simulink model "stepRecovery"  (Simulink 8.8)
settings: Solver=FixedStepDiscrete  StartTime=0.0  StopTime="CONFIG.SIMULATION_TIME "  FixedStep=CONFIG.Ts  RelTol=1e-3
InitFcn:
  | cd(fileparts(which(bdroot)));
  | initStepRecovery;
undefined symbols (not defined in the file or in its folder): bVectorConstraints, bVectorConstraintsMPC, CONFIG, ConstraintsMatrix, ConstraintsMatrixMPC, DiscIntNeverNeededParam, gain, mpc_init, reg, ROBOT_DOF, ROBOT_DOF_FOR_SIMULINK, sat, sm, WBT_robotName
libraries: WBToolboxLibrary x112, simulink x13, simulink_extras x4
(part 2 of 4)

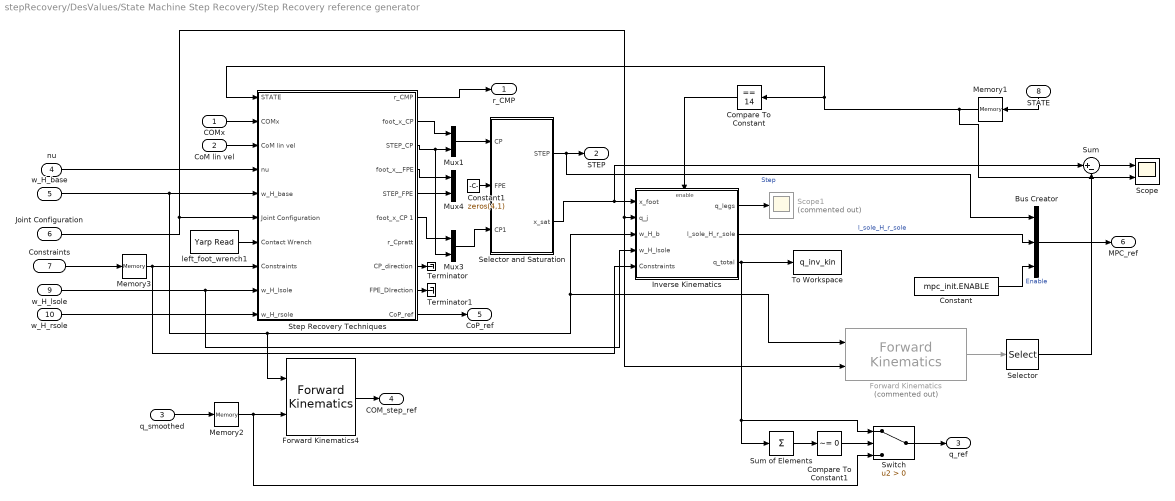
== system stepRecovery/DesValues/State Machine Step Recovery/Step Recovery reference generator ==
  COMx : Inport
  CoM lin vel : Inport  Port=2
  "q_smoothed " : Inport  Port=3
  nu : Inport  Port=4
  w_H_base : Inport  Port=5
  Joint Configuration : Inport  Port=6
  Constraints : Inport  Port=7
  STATE : Inport  Port=8
  w_H_lsole : Inport  Port=9
  w_H_rsole : Inport  Port=10
  Bus Creator : BusCreator  Inputs=3
  Compare To Constant : simulink/Logic and Bit Operations/Compare To Constant  relop===  const=14  OutDataTypeStr=boolean
  Compare To Constant1 : simulink/Logic and Bit Operations/Compare To Constant  relop=~=  const=0  OutDataTypeStr=boolean
  Constant : Constant  Value=mpc_init.ENABLE
  Constant1 : Constant  Value=zeros(4,1)
  Forward Kinematics : WBToolboxLibrary/wholeBodyModel/Kinematics/Forward Kinematics  Commented=on  frameName='r_sole'  robotName=WBT_robotName  localName=WBT_modelName  wbiFile=WBT_wbiFilename  wbiList=WBT_wbiList
  Forward Kinematics4 : WBToolboxLibrary/wholeBodyModel/Kinematics/Forward Kinematics  frameName='com'  robotName=WBT_robotName  localName=WBT_modelName  wbiFile=WBT_wbiFilename  wbiList=WBT_wbiList
  Inverse Kinematics : Subsystem  TreatAsAtomicUnit=on
  Memory1 : Memory  X0=2
  Memory2 : Memory
  Memory3 : Memory  X0=[1;1]
  Mux1 : Mux  Inputs=2
  Mux3 : Mux  Inputs=2
  Mux4 : Mux  Inputs=2
  Scope : Scope  NumInputPorts=2
  Scope1 : Scope  Commented=on
  Selector : Selector  NumberOfDimensions=2  InputPortWidth=3  IndexOptions=Index vector (dialog),Index vector (dialog)  Indices=[1:3],4  OutputSizes=1,1
  Selector and Saturation : Subsystem
  "Step Recovery Techniques " : Subsystem
  Sum : Sum  Inputs=|+-
  Sum of Elements : Sum  Inputs=+
  Switch : Switch  Criteria=u2 > Threshold
  Terminator : Terminator
  Terminator1 : Terminator
  To Workspace : ToWorkspace  VariableName=q_inv_kin  SampleTime=-1
  left_foot_wrench1 : WBToolboxLibrary/Utilities/Yarp Read  portName=PORTS.WBDT_LEFTLEG_EE  signalSize=6  blocking=off  timestamp=off  autoconnect=on  errorOnConnection=on
  r_CMP : Outport
  STEP : Outport  Port=2
  q_ref : Outport  Port=3
  COM_step_ref : Outport  Port=4
  CoP_ref : Outport  Port=5
  MPC_ref : Outport  Port=6
  wires:
  nu/1 -> "Step Recovery Techniques "/4(nu)
  Constraints/1 -> Memory3/1
  Joint Configuration/1 -> Forward Kinematics/2, Inverse Kinematics/2(q_j), "Step Recovery Techniques "/6(Joint Configuration)
  STATE/1 -> Memory1/1
  w_H_base/1 -> Forward Kinematics4/1, Forward Kinematics/1, Inverse Kinematics/3(w_H_b), "Step Recovery Techniques "/5(w_H_base)
  Selector and Saturation/1(STEP) -> Bus Creator/1, STEP/1  "Step"
  left_foot_wrench1/1 -> "Step Recovery Techniques "/7(Contact Wrench)
  "Step Recovery Techniques "/1(r_CMP) -> r_CMP/1
  Selector and Saturation/2(x_sat) -> Sum/1, Inverse Kinematics/1(x_foot)
  Inverse Kinematics/1(q_legs) -> Scope1/1
  Compare To Constant/1 -> Inverse Kinematics/Enable
  Memory1/1 -> Scope/2, "Step Recovery Techniques "/1(STATE), Compare To Constant/1
  Forward Kinematics/1 -> Selector/1
  Selector/1 -> Sum/2
  Sum/1 -> Scope/1
  Inverse Kinematics/3("q_total ") -> Switch/1, Sum of Elements/1, To Workspace/1
  "q_smoothed "/1 -> Memory2/1
  Memory2/1 -> Switch/3, Forward Kinematics4/2
  Memory3/1 -> Inverse Kinematics/5(Constraints), "Step Recovery Techniques "/8("Constraints ")
  "Step Recovery Techniques "/3(STEP_CP) -> Mux3/2, Mux1/2
  "Step Recovery Techniques "/2("foot_x_CP ") -> Mux1/1
  "Step Recovery Techniques "/6(foot_x_CP 1) -> Mux3/1
  Mux1/1 -> Selector and Saturation/1(CP)
  Mux3/1 -> Selector and Saturation/3("CP1 ")
  "Step Recovery Techniques "/4(foot_x__FPE) -> Mux4/1
  "Step Recovery Techniques "/5(STEP_FPE) -> Mux4/2
  "Step Recovery Techniques "/8(CP_direction) -> Terminator/1
  "Step Recovery Techniques "/9(FPE_DIrection) -> Terminator1/1
  w_H_lsole/1 -> "Step Recovery Techniques "/9(w_H_lsole), Inverse Kinematics/4(w_H_lsole)
  w_H_rsole/1 -> "Step Recovery Techniques "/10(w_H_rsole)
  COMx/1 -> "Step Recovery Techniques "/2(COMx)
  CoM lin vel/1 -> "Step Recovery Techniques "/3(CoM lin vel)
  Constant1/1 -> Selector and Saturation/2(FPE)
  "Step Recovery Techniques "/10("CoP_ref ") -> CoP_ref/1
  Inverse Kinematics/2(l_sole_H_r_sole) -> Bus Creator/2  "l_sole_H_r_sole"
  Bus Creator/1 -> MPC_ref/1
  Constant/1 -> Bus Creator/3  "Enable"
  Forward Kinematics4/1 -> COM_step_ref/1
  Sum of Elements/1 -> Compare To Constant1/1
  Switch/1 -> q_ref/1
  Compare To Constant1/1 -> Switch/2

== system stepRecovery/DesValues/State Machine Step Recovery/Switch ==
  Constant : Constant  Value=0
  Constant2 : Constant
  Manual Switch : ManualSwitch
  Out1 : Outport
  wires:
  Constant2/1 -> Manual Switch/2
  Manual Switch/1 -> Out1/1
  Constant/1 -> Manual Switch/1

== system stepRecovery/DesValues/State Machine Step Recovery/Visualise external wrenches   ==
  wL_WBDT : Inport
  wR_WBDT : Inport  Port=2
  CHEST_WBDT : Inport  Port=3
  Enable : EnablePort
  Constant : Constant  Value=sm.wrench.thresholdContactOn
  Constant2 : Constant  Value=sm.wrench.thresholdContactOff
  Selector : Selector  Commented=through  InputPortWidth=6  IndexOptions=Index vector (dialog)  Indices=[1:3]  OutputSizes=1
  To Workspace : ToWorkspace  VariableName=left_wrench  SampleTime=-1
  To Workspace1 : ToWorkspace  VariableName=right_wrench  SampleTime=-1
  To Workspace2 : ToWorkspace  VariableName=torso_wrench  SampleTime=-1
  chest ext wrench1 : Scope
  left foot ext wrench : Scope  NumInputPorts=3
  right foot ext wrench : Scope  NumInputPorts=3
  wires:
  Constant2/1 -> right foot ext wrench/3, left foot ext wrench/3  "thresholdContactOff"
  wL_WBDT/1 -> To Workspace/1, left foot ext wrench/1  "wL_WBDT"
  wR_WBDT/1 -> To Workspace1/1, right foot ext wrench/1  "wR_WBDT"
  Constant/1 -> right foot ext wrench/2, left foot ext wrench/2  "thresholdContactOn"
  CHEST_WBDT/1 -> To Workspace2/1, Selector/1
  Selector/1 -> chest ext wrench1/1

== system stepRecovery/DesValues/State Machine Step Recovery/Visualize hom transf5 ==
  "State " : Inport
  H : Inport  Port=2
  "CoM6D ->  CoMXYZ1" : Selector  NumberOfDimensions=2  InputPortWidth=7  IndexOptions=Index vector (dialog),Index vector (dialog)  Indices=[1 2 3],[1 2 3]  OutputSizes=1,1
  Hom : Scope  NumInputPorts=2
  MATLAB Function : MATLAB Function  TreatAsAtomicUnit=on
  p : Scope  NumInputPorts=2
  position : Selector  NumberOfDimensions=2  InputPortWidth=7  IndexOptions=Index vector (dialog),Index vector (dialog)  Indices=[1 2 3],[4]  OutputSizes=1,1
  rollPitchYaw : Scope  NumInputPorts=2
  wires:
  MATLAB Function/1(rollPitchYaw) -> rollPitchYaw/1  "rollPitchYaw"
  "CoM6D ->  CoMXYZ1"/1 -> MATLAB Function/1(R)
  H/1 -> "CoM6D ->  CoMXYZ1"/1, Hom/1, position/1  "H"
  position/1 -> p/1  "position"
  "State "/1 -> Hom/2, rollPitchYaw/2, p/2

== system stepRecovery/DesValues/State Machine Step Recovery/nu ==
  qj : Inport
  w_H_b : Inport  Port=2
  "constraints " : Inport  Port=3
  Get Estimate : WBToolboxLibrary/wholeBodyStates/Get Estimate  estimateType=Joints Velocity  robotName=WBT_robotName  localName=WBT_modelName  wbiFile=WBT_wbiFilename  wbiList=WBT_wbiList
  Jacobian l_sole : WBToolboxLibrary/wholeBodyModel/Jacobians/Jacobian  frameName='l_sole'  robotName=WBT_robotName  localName=WBT_modelName  wbiFile=WBT_wbiFilename  wbiList=WBT_wbiList
  Jacobian r_sole : WBToolboxLibrary/wholeBodyModel/Jacobians/Jacobian  frameName='r_sole'  robotName=WBT_robotName  localName=WBT_modelName  wbiFile=WBT_wbiFilename  wbiList=WBT_wbiList
  MATLAB Function : MATLAB Function  TreatAsAtomicUnit=on
  Mux : Mux  Inputs=2
  vb + Dqj : Outport
  wires:
  w_H_b/1 -> Jacobian l_sole/1, Jacobian r_sole/1
  qj/1 -> Jacobian l_sole/2, Jacobian r_sole/2
  Jacobian l_sole/1 -> MATLAB Function/1(JcLeftFoot)
  MATLAB Function/1(y) -> Mux/1
  "constraints "/1 -> MATLAB Function/3(activeFeetConstraints)
  Jacobian r_sole/1 -> MATLAB Function/2(JcRightFoot)
  Mux/1 -> vb + Dqj/1
  Get Estimate/1 -> Mux/2, MATLAB Function/4(qD)

== system stepRecovery/DesValues/State Machine Step Recovery/visualise inertial ==
  jointAngles : Inport
  inertial : Inport  Port=2
  Enable : EnablePort
  Inv\* : Product  Inputs=/*  Multiplication=Matrix(*)
  Inv\*1 : Product  Inputs=/*  Multiplication=Matrix(*)
  Visualize hom transf1 : Subsystem
  Visualize hom transf2 : Subsystem
  Visualize hom transf3 : Subsystem
  Visualize hom transf4 : Subsystem
  Visualize hom transf5 : Subsystem
  Visualize hom transf6 : Subsystem
  "inertial -> rpy" : Selector  InputPortWidth=12  IndexOptions=Index vector (dialog)  Indices=[1 2 3]  OutputSizes=1
  l_sole_H_root_link2 : Subsystem  mask{link_name='l_sole'}
  l_sole_H_root_link3 : Subsystem  mask{link_name='r_sole'}
  rpy : Scope
  w_H_root_link1 : Subsystem  mask{link_name='r_sole'}
      mask prompts: link_name "link name"
      mask help:
      | This block evaluates the homogeneous transformation between the world and the root link, i.e. ^wH_b. It assumes that the link specified by the variable 'link_name' has a constant position
      | w.r.t. an inertial frame, but it can rotate arbitrarily. This rotation is retrived from the IMU sensor.
      mask Display:
      | str = strrep(link_name, '_','\_');
      | port_label('output',1,['{}^{',str '}H_{root}'],'texmode','on')
      | clear str;
      | 
      | port_label('input',1,'q_j','texmode','on')
      | 
      | port_label('input',2,'inertial','texmode','on')
  w_H_root_link4 : Subsystem  mask{link_name='l_sole'}
      mask prompts: link_name "link name"
      mask help:
      | This block evaluates the homogeneous transformation between the world and the root link, i.e. ^wH_b. It assumes that the link specified by the variable 'link_name' has a constant position
      | w.r.t. an inertial frame, but it can rotate arbitrarily. This rotation is retrived from the IMU sensor.
      mask Display:
      | str = strrep(link_name, '_','\_');
      | port_label('output',1,['{}^{',str '}H_{root}'],'texmode','on')
      | clear str;
      | 
      | port_label('input',1,'q_j','texmode','on')
      | 
      | port_label('input',2,'inertial','texmode','on')
  wires:
  w_H_root_link1/1(w_H_root) -> Inv\*1/2, Visualize hom transf3/1(H)
  Inv\*1/1 -> Visualize hom transf1/1(H)
  l_sole_H_root_link3/1(link_name_H_root_link) -> Inv\*1/1, Visualize hom transf2/1(H)  "r_sole_H_root_link"
  "inertial -> rpy"/1 -> rpy/1
  w_H_root_link4/1(w_H_root) -> Inv\*/2, Visualize hom transf4/1(H)
  Inv\*/1 -> Visualize hom transf5/1(H)
  l_sole_H_root_link2/1(link_name_H_root_link) -> Inv\*/1, Visualize hom transf6/1(H)  "l_sole_H_root_link"
  jointAngles/1 -> l_sole_H_root_link3/1(qj), w_H_root_link1/1(qj), w_H_root_link4/1(qj), l_sole_H_root_link2/1(qj)
  inertial/1 -> w_H_root_link4/2(inertial), w_H_root_link1/2(inertial), "inertial -> rpy"/1

== system stepRecovery/DesValues/State Machine Step Recovery/w_H_root_link1 ==
  qj : Inport
  inertial : Inport  Port=2
  "CoM6D ->  CoMXYZ1" : Selector  NumberOfDimensions=2  InputPortWidth=7  IndexOptions=Index vector (dialog),Index vector (dialog)  Indices=[1 2 3],[1 2 3]  OutputSizes=1,1
  Constant : Constant  Value=zeros(3,1)
  Constant2 : Constant  Value=eye(4)
  Constant5 : Constant  Value=eye(4)
  Constant6 : Constant  Value=eye(4)
  Gain : Gain  Gain=pi/180
  Head state : WBToolboxLibrary/Utilities/Yarp Read  portName=[WBT_robotName, '/head/state:o']  signalSize=6  blocking=off  timestamp=off  autoconnect=on  errorOnConnection=off
  Inv\* : Product  Inputs=/*  Multiplication=Matrix(*)
  Inv\*1 : Product  Inputs=/*  Multiplication=Matrix(*)
  Inv\*2 : Product  Inputs=/  Multiplication=Matrix(*)
  Product : Product  Multiplication=Matrix(*)
  Selector : Selector  InputPortWidth=12  IndexOptions=Index vector (dialog)  Indices=[4 5 6 ]  OutputSizes=1
  Selector1 : Selector  InputPortWidth=6  IndexOptions=Index vector (dialog)  Indices=[1:3]  OutputSizes=1
  Switch : Switch  Criteria=u2 > Threshold
  Switch6 : Switch  Criteria=u2 > Threshold
  USE_IMU4EST_BASE : Constant  Value=CONFIG.USE_IMU4EST_BASE
  USE_IMU4EST_BASE1 : Constant  Value=CONFIG.CORRECT_NECK_IMU
  fromImuToHomogeousTransformFCN : MATLAB Function  TreatAsAtomicUnit=on
  holder 1 : WBToolboxLibrary/Utilities/holder 
  holder 2 : WBToolboxLibrary/Utilities/holder 
  imu : WBToolboxLibrary/wholeBodyModel/Kinematics/Forward Kinematics  frameName='imu_frame'  robotName=WBT_robotName  localName=WBT_modelName  wbiFile=WBT_wbiFilename  wbiList=WBT_wbiList
  l_sole_acc : Scope
  link : WBToolboxLibrary/wholeBodyModel/Kinematics/Forward Kinematics  frameName=link_name  robotName=WBT_robotName  localName=WBT_modelName  wbiFile=WBT_wbiFilename  wbiList=WBT_wbiList
  root_link : WBToolboxLibrary/wholeBodyModel/Kinematics/Forward Kinematics  frameName='root_link'  robotName=WBT_robotName  localName=WBT_modelName  wbiFile=WBT_wbiFilename  wbiList=WBT_wbiList
  w_H_root : Outport
  wires:
  Constant/1 -> Switch/3
  Gain/1 -> Selector1/1
  Switch/1 -> fromImuToHomogeousTransformFCN/6(neck)
  USE_IMU4EST_BASE1/1 -> Switch/2
  Selector1/1 -> Switch/1  "neck"
  Head state/1 -> Gain/1
  Product/1 -> l_sole_acc/1
  Selector/1 -> Product/2  "imu_acce"
  "CoM6D ->  CoMXYZ1"/1 -> Product/1  "l_sole_R_imu"
  Inv\*2/1 -> "CoM6D ->  CoMXYZ1"/1
  holder 2/1 -> fromImuToHomogeousTransformFCN/4(inertial_0)
  holder 1/1 -> fromImuToHomogeousTransformFCN/2(imu_H_link_0)
  root_link/1 -> Inv\*1/2
  qj/1 -> imu/2, link/2, root_link/2
  Constant2/1 -> root_link/1
  fromImuToHomogeousTransformFCN/1(w_H_root) -> Switch6/1
  USE_IMU4EST_BASE/1 -> Switch6/2
  Switch6/1 -> w_H_root/1
  inertial/1 -> fromImuToHomogeousTransformFCN/5(inertial), holder 2/1, Selector/1
  link/1 -> Inv\*1/1, Inv\*/2
  Inv\*1/1 -> fromImuToHomogeousTransformFCN/3(link_H_root), Switch6/3  "link_H_root"
  Constant6/1 -> link/1
  imu/1 -> Inv\*/1
  Inv\*/1 -> fromImuToHomogeousTransformFCN/1(imu_H_link), holder 1/1, Inv\*2/1  "imu_H_link"
  Constant5/1 -> imu/1

== system stepRecovery/DesValues/State Machine Step Recovery/w_H_root_link4 ==
  qj : Inport
  inertial : Inport  Port=2
  "CoM6D ->  CoMXYZ1" : Selector  NumberOfDimensions=2  InputPortWidth=7  IndexOptions=Index vector (dialog),Index vector (dialog)  Indices=[1 2 3],[1 2 3]  OutputSizes=1,1
  Constant : Constant  Value=zeros(3,1)
  Constant2 : Constant  Value=eye(4)
  Constant5 : Constant  Value=eye(4)
  Constant6 : Constant  Value=eye(4)
  Gain : Gain  Gain=pi/180
  Head state : WBToolboxLibrary/Utilities/Yarp Read  portName=[WBT_robotName, '/head/state:o']  signalSize=6  blocking=off  timestamp=off  autoconnect=on  errorOnConnection=off
  Inv\* : Product  Inputs=/*  Multiplication=Matrix(*)
  Inv\*1 : Product  Inputs=/*  Multiplication=Matrix(*)
  Inv\*2 : Product  Inputs=/  Multiplication=Matrix(*)
  Product : Product  Multiplication=Matrix(*)
  Selector : Selector  InputPortWidth=12  IndexOptions=Index vector (dialog)  Indices=[4 5 6 ]  OutputSizes=1
  Selector1 : Selector  InputPortWidth=6  IndexOptions=Index vector (dialog)  Indices=[1:3]  OutputSizes=1
  Switch : Switch  Criteria=u2 > Threshold
  Switch6 : Switch  Criteria=u2 > Threshold
  USE_IMU4EST_BASE : Constant  Value=CONFIG.USE_IMU4EST_BASE
  USE_IMU4EST_BASE1 : Constant  Value=CONFIG.CORRECT_NECK_IMU
  fromImuToHomogeousTransformFCN : MATLAB Function  TreatAsAtomicUnit=on
  holder 1 : WBToolboxLibrary/Utilities/holder 
  holder 2 : WBToolboxLibrary/Utilities/holder 
  imu : WBToolboxLibrary/wholeBodyModel/Kinematics/Forward Kinematics  frameName='imu_frame'  robotName=WBT_robotName  localName=WBT_modelName  wbiFile=WBT_wbiFilename  wbiList=WBT_wbiList
  l_sole_acc : Scope
  link : WBToolboxLibrary/wholeBodyModel/Kinematics/Forward Kinematics  frameName=link_name  robotName=WBT_robotName  localName=WBT_modelName  wbiFile=WBT_wbiFilename  wbiList=WBT_wbiList
  root_link : WBToolboxLibrary/wholeBodyModel/Kinematics/Forward Kinematics  frameName='root_link'  robotName=WBT_robotName  localName=WBT_modelName  wbiFile=WBT_wbiFilename  wbiList=WBT_wbiList
  w_H_root : Outport
  wires:
  Constant/1 -> Switch/3
  Gain/1 -> Selector1/1
  Switch/1 -> fromImuToHomogeousTransformFCN/6(neck)
  USE_IMU4EST_BASE1/1 -> Switch/2
  Selector1/1 -> Switch/1  "neck"
  Head state/1 -> Gain/1
  Product/1 -> l_sole_acc/1
  Selector/1 -> Product/2  "imu_acce"
  "CoM6D ->  CoMXYZ1"/1 -> Product/1  "l_sole_R_imu"
  Inv\*2/1 -> "CoM6D ->  CoMXYZ1"/1
  holder 2/1 -> fromImuToHomogeousTransformFCN/4(inertial_0)
  holder 1/1 -> fromImuToHomogeousTransformFCN/2(imu_H_link_0)
  root_link/1 -> Inv\*1/2
  qj/1 -> imu/2, link/2, root_link/2
  Constant2/1 -> root_link/1
  fromImuToHomogeousTransformFCN/1(w_H_root) -> Switch6/1
  USE_IMU4EST_BASE/1 -> Switch6/2
  Switch6/1 -> w_H_root/1
  inertial/1 -> fromImuToHomogeousTransformFCN/5(inertial), holder 2/1, Selector/1
  link/1 -> Inv\*1/1, Inv\*/2
  Inv\*1/1 -> fromImuToHomogeousTransformFCN/3(link_H_root), Switch6/3  "link_H_root"
  Constant6/1 -> link/1
  imu/1 -> Inv\*/1
  Inv\*/1 -> fromImuToHomogeousTransformFCN/1(imu_H_link), holder 1/1, Inv\*2/1  "imu_H_link"
  Constant5/1 -> imu/1

== system stepRecovery/DesValues/State Machine Step Recovery/xCom ==
  qj : Inport
  w_H_b : Inport  Port=2
  "CoM6D ->  CoMXYZ2" : Selector  NumberOfDimensions=2  InputPortWidth=7  IndexOptions=Index vector (dialog),Index vector (dialog)  Indices=[1 2 3],[4]  OutputSizes=1,1
  com : WBToolboxLibrary/wholeBodyModel/Kinematics/Forward Kinematics  frameName='com'  robotName=WBT_robotName  localName=WBT_modelName  wbiFile=WBT_wbiFilename  wbiList=WBT_wbiList
  xCom : Outport
  wires:
  w_H_b/1 -> com/1
  com/1 -> "CoM6D ->  CoMXYZ2"/1
  "CoM6D ->  CoMXYZ2"/1 -> xCom/1
  qj/1 -> com/2

== system stepRecovery/DesValues/State Machine Step Recovery/xCom1 ==
  qj : Inport
  w_H_b : Inport  Port=2
  "CoM6D ->  CoMXYZ2" : Selector  NumberOfDimensions=2  InputPortWidth=7  IndexOptions=Index vector (dialog),Index vector (dialog)  Indices=[1 2 3],[4]  OutputSizes=1,1
  com : WBToolboxLibrary/wholeBodyModel/Kinematics/Forward Kinematics  frameName='com'  robotName=WBT_robotName  localName=WBT_modelName  wbiFile=WBT_wbiFilename  wbiList=WBT_wbiList
  xCom : Outport
  wires:
  w_H_b/1 -> com/1
  com/1 -> "CoM6D ->  CoMXYZ2"/1
  "CoM6D ->  CoMXYZ2"/1 -> xCom/1
  qj/1 -> com/2

== system stepRecovery/controller_QP/MPC /omega ==
  COMx : Inport
  Constant : Constant  Value=9.81
  Divide : Product  Inputs=*/
  Selector : Selector  InputPortWidth=3  IndexOptions=Index vector (dialog)  Indices=[3]  OutputSizes=1
  Sqrt : Sqrt  SaturateOnIntegerOverflow=on
  holder 1 : WBToolboxLibrary/Utilities/holder 
  COMz0 : Outport
  omega : Outport  Port=2
  wires:
  COMx/1 -> Selector/1
  Selector/1 -> holder 1/1
  holder 1/1 -> COMz0/1, Divide/2
  Constant/1 -> Divide/1
  Divide/1 -> Sqrt/1
  Sqrt/1 -> omega/1

== system stepRecovery/controller_QP/QP/Subsystem ==
  LEFT_RIGHT_FOOT_IN_CONTACT : Inport
  HessianMatrixQP2Feet : Inport  Port=2
  gradientQP2Feet : Inport  Port=3
  ConstraintsMatrixQP2Feet : Inport  Port=4
  bVectorConstraintsQp2Feet : Inport  Port=5
  USE_QP : Inport  Port=6
  HessianMatrixQP1Foot : Inport  Port=7
  gradientQP1Foot : Inport  Port=8
  ConstraintsMatrixQP1Foot : Inport  Port=9
  bVectorConstraintsQP1Foot : Inport  Port=10
  Enable : EnablePort
  Level-2 MATLAB S-Function : M-S-Function  FunctionName=QpBalancing
  f0TwoFeet : Outport
  ExitFlag : Outport  Port=2
  f0OneFoot : Outport  Port=3
  wires:
  Level-2 MATLAB S-Function/1 -> f0TwoFeet/1
  Level-2 MATLAB S-Function/2 -> ExitFlag/1  "Exit flag QP two feet"
  HessianMatrixQP1Foot/1 -> Level-2 MATLAB S-Function/7
  bVectorConstraintsQP1Foot/1 -> Level-2 MATLAB S-Function/10
  gradientQP1Foot/1 -> Level-2 MATLAB S-Function/8
  ConstraintsMatrixQP1Foot/1 -> Level-2 MATLAB S-Function/9
  Level-2 MATLAB S-Function/3 -> f0OneFoot/1
  LEFT_RIGHT_FOOT_IN_CONTACT/1 -> Level-2 MATLAB S-Function/1
  HessianMatrixQP2Feet/1 -> Level-2 MATLAB S-Function/2
  gradientQP2Feet/1 -> Level-2 MATLAB S-Function/3
  ConstraintsMatrixQP2Feet/1 -> Level-2 MATLAB S-Function/4
  bVectorConstraintsQp2Feet/1 -> Level-2 MATLAB S-Function/5
  USE_QP/1 -> Level-2 MATLAB S-Function/6

== system stepRecovery/controller_QP/QP/Subsystem1 ==
  LEFT_RIGHT_FOOT_IN_CONTACT : Inport
  HessianMatrixQP2Feet : Inport  Port=2
  gradientQP2Feet : Inport  Port=3
  ConstraintsMatrixQP2Feet : Inport  Port=4
  bVectorConstraintsQp2Feet : Inport  Port=5
  USE_QP : Inport  Port=6
  HessianMatrixQP1Foot : Inport  Port=7
  gradientQP1Foot : Inport  Port=8
  ConstraintsMatrixQP1Foot : Inport  Port=9
  bVectorConstraintsQP1Foot : Inport  Port=10
  Enable : EnablePort
  Level-2 MATLAB S-Function : M-S-Function  FunctionName=QpTwoFeetStep
  f0TwoFeet : Outport
  ExitFlag : Outport  Port=2
  f0OneFoot : Outport  Port=3
  slack : Outport  Port=4
  wires:
  USE_QP/1 -> Level-2 MATLAB S-Function/6
  bVectorConstraintsQp2Feet/1 -> Level-2 MATLAB S-Function/5
  ConstraintsMatrixQP2Feet/1 -> Level-2 MATLAB S-Function/4
  gradientQP2Feet/1 -> Level-2 MATLAB S-Function/3
  HessianMatrixQP2Feet/1 -> Level-2 MATLAB S-Function/2
  LEFT_RIGHT_FOOT_IN_CONTACT/1 -> Level-2 MATLAB S-Function/1
  Level-2 MATLAB S-Function/3 -> f0OneFoot/1
  ConstraintsMatrixQP1Foot/1 -> Level-2 MATLAB S-Function/9
  gradientQP1Foot/1 -> Level-2 MATLAB S-Function/8
  bVectorConstraintsQP1Foot/1 -> Level-2 MATLAB S-Function/10
  HessianMatrixQP1Foot/1 -> Level-2 MATLAB S-Function/7
  Level-2 MATLAB S-Function/2 -> ExitFlag/1  "Exit flag QP two feet"
  Level-2 MATLAB S-Function/1 -> f0TwoFeet/1
  Level-2 MATLAB S-Function/4 -> slack/1

== system stepRecovery/controller_QP/QP/Visualize eventual QP failures ==
  exitFlagQP : Inport
  state : Inport  Port=2
  Enable : EnablePort
  "QP status (0: no failure, 1: not using)" : Scope  NumInputPorts=2
  wires:
  exitFlagQP/1 -> "QP status (0: no failure, 1: not using)"/1  "exitFlagQP"
  state/1 -> "QP status (0: no failure, 1: not using)"/2

== system stepRecovery/controller_QP/integralOf Hw/l_sole_H_root_link ==
  qj0 : Inport
  Constant5 : Constant  Value=eye(4)
  Constant6 : Constant  Value=eye(4)
  Inv\* : Product  Inputs=/*  Multiplication=Matrix(*)
  l_sole : WBToolboxLibrary/wholeBodyModel/Kinematics/Forward Kinematics  frameName='l_sole'  robotName=WBT_robotName  localName=WBT_modelName  wbiFile=WBT_wbiFilename  wbiList=WBT_wbiList
  root_link : WBToolboxLibrary/wholeBodyModel/Kinematics/Forward Kinematics  frameName='root_link'  robotName=WBT_robotName  localName=WBT_modelName  wbiFile=WBT_wbiFilename  wbiList=WBT_wbiList
  l_sole_H_root_link : Outport
  wires:
  Constant5/1 -> l_sole/1
  Inv\*/1 -> l_sole_H_root_link/1  "l_sole_H_root_link"
  l_sole/1 -> Inv\*/1
  Constant6/1 -> root_link/1
  qj0/1 -> l_sole/2, root_link/2
  root_link/1 -> Inv\*/2

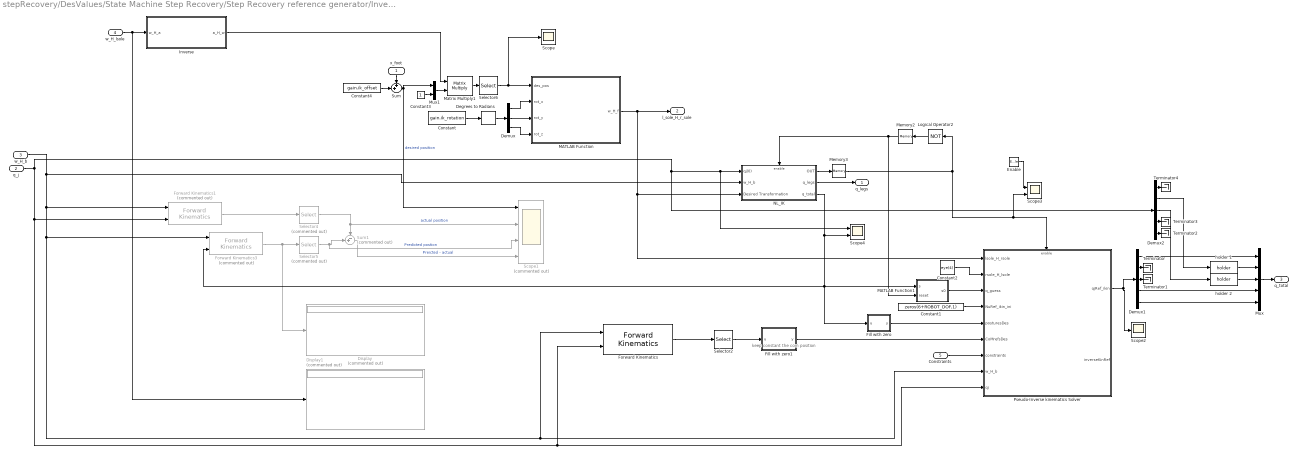
== system stepRecovery/DesValues/State Machine Step Recovery/Step Recovery reference generator/Inverse Kinematics ==
  note: keep constant the com position
  x_foot : Inport
  q_j : Inport  Port=2
  w_H_b : Inport  Port=3
  w_H_lsole : Inport  Port=4
  Constraints : Inport  Port=5
  Enable : EnablePort  ShowOutputPort=on
  Constant : Constant  Value=gain.ik_rotation
  Constant1 : Constant  Value=zeros(6+ROBOT_DOF,1)
  Constant2 : Constant  Value=eye(4)
  Constant3 : Constant
  Constant4 : Constant  Value=gain.ik_offset
  Degrees to Radians : simulink_extras/Transformations/Degrees to Radians
  Demux : Demux  Outputs=3
  Demux1 : Demux  Outputs=[3;4;4;6;6]
  Demux2 : Demux  Outputs=[3;4;4;6;6]
  Display : Display  Commented=on
  Display1 : Display  Commented=on
  Fill with zero : MATLAB Function  TreatAsAtomicUnit=on
  Fill with zero1 : MATLAB Function  TreatAsAtomicUnit=on
  Forward Kinematics : WBToolboxLibrary/wholeBodyModel/Kinematics/Forward Kinematics  frameName='com'  robotName=WBT_robotName  localName=WBT_modelName  wbiFile=WBT_wbiFilename  wbiList=WBT_wbiList
  Forward Kinematics1 : WBToolboxLibrary/wholeBodyModel/Kinematics/Forward Kinematics  Commented=on  frameName='r_sole'  robotName=WBT_robotName  localName=WBT_modelName  wbiFile=WBT_wbiFilename  wbiList=WBT_wbiList
  Forward Kinematics3 : WBToolboxLibrary/wholeBodyModel/Kinematics/Forward Kinematics  Commented=on  frameName='r_sole'  robotName=WBT_robotName  localName=WBT_modelName  wbiFile=WBT_wbiFilename  wbiList=WBT_wbiList
  Inverse : MATLAB Function  TreatAsAtomicUnit=on
  Logical Operator2 : Logic  Operator=NOT  AllPortsSameDT=off  OutDataTypeStr=boolean
  MATLAB Function : MATLAB Function  TreatAsAtomicUnit=on
  MATLAB Function1 : MATLAB Function  TreatAsAtomicUnit=on
  Matrix Multiply1 : Product  Multiplication=Matrix(*)
  Memory2 : Memory  X0=1
  Memory3 : Memory
  Mux : Mux  Inputs=[3;4;4;6;6]
  Mux1 : Mux  Inputs=2
  NL_IK : Subsystem
  Pseudo-Inverse kinematics Solver : Subsystem
  Scope : Scope
  Scope1 : Scope  Commented=on  NumInputPorts=4
  Scope2 : Scope
  Scope3 : Scope  NumInputPorts=2
  Scope4 : Scope  NumInputPorts=2
  Selector2 : Selector  NumberOfDimensions=2  InputPortWidth=3  IndexOptions=Index vector (dialog),Index vector (dialog)  Indices=[1:3],4  OutputSizes=1,1
  Selector4 : Selector  Commented=on  NumberOfDimensions=2  InputPortWidth=4  IndexOptions=Index vector (dialog),Index vector (dialog)  Indices=[1:3],4  OutputSizes=1,1
  Selector5 : Selector  Commented=on  NumberOfDimensions=2  InputPortWidth=4  IndexOptions=Index vector (dialog),Index vector (dialog)  Indices=[1:3],4  OutputSizes=1,1
  Selector6 : Selector  InputPortWidth=4  IndexOptions=Index vector (dialog)  Indices=[1:3]  OutputSizes=1
  Sum : Sum  Inputs=++|
  Sum1 : Sum  Commented=on  Inputs=-+|
  Terminator{,1..4} (5 alike) : Terminator
  holder 1 : WBToolboxLibrary/Utilities/holder 
  holder 2 : WBToolboxLibrary/Utilities/holder 
  q_legs : Outport
  l_sole_H_r_sole : Outport  Port=2
  "q_total " : Outport  Port=3
  wires:
  w_H_lsole/1 -> Display1/1, Inverse/1(w_H_a)
  Inverse/1(a_H_w) -> Matrix Multiply1/1
  Forward Kinematics1/1 -> Selector4/1
  Sum/1 -> Mux1/1, Scope1/1  "desired position"
  Constant4/1 -> Sum/2
  x_foot/1 -> Sum/1
  Forward Kinematics3/1 -> Display/1, Selector5/1
  Selector4/1 -> Sum1/1, Scope1/2  "actual position"
  Sum1/1 -> Scope1/4  "Preicted - actual"
  Mux1/1 -> Matrix Multiply1/2
  Constant3/1 -> Mux1/2
  Selector6/1 -> Scope/1, MATLAB Function/1(des_pos)
  Matrix Multiply1/1 -> Selector6/1
  Selector5/1 -> Scope1/3, Sum1/2  "Predicted postion"
  Constant/1 -> Degrees to Radians/1
  Degrees to Radians/1 -> Demux/1
  Demux/2 -> MATLAB Function/3(rot_y)
  Demux/1 -> MATLAB Function/2(rot_x)
  Demux/3 -> MATLAB Function/4(rot_z)
  MATLAB Function/1(w_H_f) -> l_sole_H_r_sole/1, Pseudo-Inverse kinematics Solver/1("lsole_H_rsole "), NL_IK/3(Desired Transformation)
  w_H_b/1 -> NL_IK/2(w_H_b), Forward Kinematics1/1, Forward Kinematics/1, Pseudo-Inverse kinematics Solver/8("w_H_b "), Forward Kinematics3/1
  Constant1/1 -> Pseudo-Inverse kinematics Solver/4(NuRef_ikin_ini)
  Constraints/1 -> Pseudo-Inverse kinematics Solver/7(constraints)
  Fill with zero1/1(y) -> Pseudo-Inverse kinematics Solver/6(CoMrefsDes)
  Forward Kinematics/1 -> Selector2/1
  Selector2/1 -> Fill with zero1/1(u)
  Fill with zero/1(y) -> Pseudo-Inverse kinematics Solver/5(posturesDes)
  MATLAB Function1/1(s0) -> Pseudo-Inverse kinematics Solver/3(q_guess)
  Logical Operator2/1 -> Memory2/1
  q_j/1 -> Forward Kinematics/2, Pseudo-Inverse kinematics Solver/9(qj), Forward Kinematics1/2, Demux2/1, Scope4/1, NL_IK/1(qj(0))
  Demux1/1 -> Mux/1
  Demux1/4 -> Mux/4
  Demux1/5 -> Mux/5
  Demux1/2 -> Terminator/1
  Demux1/3 -> Terminator1/1
  holder 2/1 -> Mux/3
  holder 1/1 -> Mux/2
  Demux2/2 -> holder 1/1
  Demux2/3 -> holder 2/1
  Demux2/5 -> Terminator2/1
  Demux2/4 -> Terminator3/1
  Demux2/1 -> Terminator4/1
  Memory2/1 -> NL_IK/Enable, MATLAB Function1/2(reset)
  Enable/1 -> Scope3/1
  Memory3/1 -> Pseudo-Inverse kinematics Solver/Enable, Scope3/2, Logical Operator2/1
  Mux/1 -> "q_total "/1
  NL_IK/2(q_legs) -> q_legs/1
  NL_IK/1(OUT) -> Memory3/1
  Constant2/1 -> Pseudo-Inverse kinematics Solver/2(rsole_H_lsole)
  NL_IK/3(q_total) -> Forward Kinematics3/2, MATLAB Function1/1(s), Fill with zero/1(u), Scope4/2
  Pseudo-Inverse kinematics Solver/1(qjRef_ikin) -> Scope2/1, Demux1/1

== system stepRecovery/DesValues/State Machine Step Recovery/Step Recovery reference generator/Selector and Saturation ==
  CP : Inport
  FPE : Inport  Port=2
  "CP1 " : Inport  Port=3
  Constant : Constant  Value=2*sqrt(gain.leg_length^2 - gain.minimum_height^2)
  Constant1 : Constant  Value=gain.min_step_length
  Constant2 : Constant  Value=CONFIG.SR.TECHNIQUE
  Demux : Demux
  Dot Product : DotProduct  InputSameDT=on  OutDataTypeStr=Inherit: Inherit via internal rule
  MATLAB Function : MATLAB Function  TreatAsAtomicUnit=on
  Multiport Switch : MultiPortSwitch  DataPortOrder=Specify indices  DataPortIndices={2,1,0}
  Mux : Mux  Inputs=3
  Mux1 : Mux  Inputs=3
  Scope : Scope  Commented=on  NumInputPorts=4
  Sqrt : Sqrt  SaturateOnIntegerOverflow=on
  To Workspace : ToWorkspace  VariableName=IS_SATURATED  SampleTime=-1
      settings: Save2DSignal=2-D array (concatenate along first dimension)
  STEP : Outport
  x_sat : Outport  Port=2
  wires:
  Mux1/1 -> Scope/4, Dot Product/2, Dot Product/1, MATLAB Function/1(x)  "X"
  Constant/1 -> MATLAB Function/2(max_d), Mux/2  "max module"
  MATLAB Function/1(x_sat) -> Scope/3, x_sat/1  "X_SAT"
  MATLAB Function/2(SAT) -> Scope/1, To Workspace/1  "SAT"
  Mux/1 -> Scope/2  "MODULE"
  Sqrt/1 -> Mux/1  "desired module"
  Dot Product/1 -> Sqrt/1
  Constant1/1 -> Mux/3, MATLAB Function/3(min_d)  "min module"
  Multiport Switch/1 -> Demux/1  "X"
  Demux/4 -> STEP/1
  CP/1 -> Multiport Switch/4  "X"
  FPE/1 -> Multiport Switch/3
  "CP1 "/1 -> Multiport Switch/2
  Constant2/1 -> Multiport Switch/1
  Demux/2 -> Mux1/2
  Demux/3 -> Mux1/3
  Demux/1 -> Mux1/1  "X"

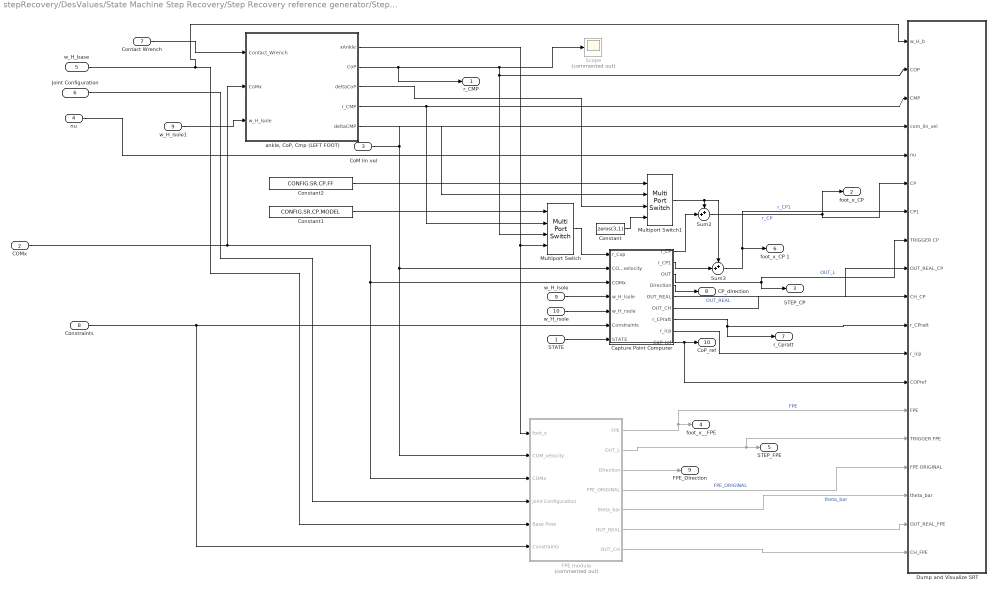
== system stepRecovery/DesValues/State Machine Step Recovery/Step Recovery reference generator/Step Recovery Techniques  ==
  STATE : Inport
  COMx : Inport  Port=2
  CoM lin vel : Inport  Port=3
  nu : Inport  Port=4
  w_H_base : Inport  Port=5
  Joint Configuration : Inport  Port=6
  Contact Wrench : Inport  Port=7
  "Constraints " : Inport  Port=8
  w_H_lsole : Inport  Port=9
  w_H_rsole : Inport  Port=10
  Capture Point Computer : Subsystem
  Constant : Constant  Value=zeros(3,1)
  Constant1 : Constant  Value=CONFIG.SR.CP.MODEL
  Constant2 : Constant  Value=CONFIG.SR.CP.FF
  "Dump and Visualize SRT " : Subsystem
  FPE module : Subsystem  Commented=on
  Multiport Switch : MultiPortSwitch  DataPortOrder=Specify indices  DataPortIndices={2,1,0}
  Multiport Switch1 : MultiPortSwitch  DataPortOrder=Specify indices  DataPortIndices={2,1,0}
  Scope : Scope  Commented=on
  Sum2 : Sum  Inputs=++|
  Sum3 : Sum  Inputs=++|
  "ankle, CoP, Cmp (LEFT FOOT)" : Subsystem
  w_H_lsole1 : InportShadow  Port=9
  r_CMP : Outport
  "foot_x_CP " : Outport  Port=2
  STEP_CP : Outport  Port=3
  foot_x__FPE : Outport  Port=4
  STEP_FPE : Outport  Port=5
  foot_x_CP 1 : Outport  Port=6
  "r_Cpratt " : Outport  Port=7
  CP_direction : Outport  Port=8
  FPE_DIrection : Outport  Port=9
  "CoP_ref " : Outport  Port=10
  wires:
  Joint Configuration/1 -> FPE module/4(Joint Configuration)
  w_H_base/1 -> FPE module/5(Base Pose), "Dump and Visualize SRT "/1(w_H_b)
  FPE module/1(FPE) -> "Dump and Visualize SRT "/14(FPE), foot_x__FPE/1  "FPE"
  Sum2/1 -> "foot_x_CP "/1, "Dump and Visualize SRT "/6(CP)  "r_CP"
  Capture Point Computer/3(OUT) -> "Dump and Visualize SRT "/8(TRIGGER CP), STEP_CP/1  "OUT_L"
  Sum3/1 -> "Dump and Visualize SRT "/7(CP1), foot_x_CP 1/1  "r_CP1"
  FPE module/3(Direction) -> FPE_DIrection/1
  Capture Point Computer/4(Direction) -> CP_direction/1
  Capture Point Computer/1(r_CP) -> Sum2/2
  Capture Point Computer/2(r_CP1) -> Sum3/2
  "Constraints "/1 -> FPE module/6(Constraints), Capture Point Computer/6("Constraints ")
  FPE module/2(OUT_L) -> "Dump and Visualize SRT "/15(TRIGGER FPE), STEP_FPE/1
  CoM lin vel/1 -> "Dump and Visualize SRT "/4(com_lin_vel), FPE module/2(COM_velocity), Capture Point Computer/2(COM velocity)
  COMx/1 -> FPE module/3(COMx), Capture Point Computer/3(COMx), "ankle, CoP, Cmp (LEFT FOOT)"/2(CoMx)
  "ankle, CoP, Cmp (LEFT FOOT)"/2(CoP) -> r_CMP/1, Scope/1, Multiport Switch/3, "Dump and Visualize SRT "/2(COP)
  "ankle, CoP, Cmp (LEFT FOOT)"/1(xAnkle) -> FPE module/1(foot_x), Multiport Switch/4
  Contact Wrench/1 -> "ankle, CoP, Cmp (LEFT FOOT)"/1(Contact_Wrench)
  nu/1 -> "Dump and Visualize SRT "/5(nu)
  "ankle, CoP, Cmp (LEFT FOOT)"/4(r_CMP) -> "Dump and Visualize SRT "/3(CMP), Multiport Switch/2
  Capture Point Computer/5(OUT_REAL) -> "Dump and Visualize SRT "/9(OUT_REAL_CP)  "OUT_REAL"
  Capture Point Computer/6(OUT_CH) -> "Dump and Visualize SRT "/10(CH_CP)
  FPE module/4(FPE_ORIGINAL) -> "Dump and Visualize SRT "/16(FPE ORIGINAL)  "FPE_ORIGINAL"
  FPE module/5(theta_bar) -> "Dump and Visualize SRT "/17(theta_bar)  "theta_bar"
  FPE module/6(OUT_REAL) -> "Dump and Visualize SRT "/18(OUT_REAL_FPE)
  FPE module/7(OUT_CH) -> "Dump and Visualize SRT "/19(CH_FPE)
  Multiport Switch/1 -> Capture Point Computer/1(r_Cxp)
  Multiport Switch1/1 -> Sum3/1, Sum2/1
  Constant/1 -> Multiport Switch1/4
  "ankle, CoP, Cmp (LEFT FOOT)"/3(deltaCoP) -> Multiport Switch1/3
  "ankle, CoP, Cmp (LEFT FOOT)"/5(deltaCMP) -> Multiport Switch1/2
  Constant1/1 -> Multiport Switch/1
  Constant2/1 -> Multiport Switch1/1
  w_H_lsole/1 -> Capture Point Computer/4(w_H_lsole)
  w_H_rsole/1 -> Capture Point Computer/5(w_H_rsole)
  w_H_lsole1/1 -> "ankle, CoP, Cmp (LEFT FOOT)"/3(w_H_lsole)
  STATE/1 -> Capture Point Computer/7(STATE)
  Capture Point Computer/7("r_CPratt ") -> "r_Cpratt "/1, "Dump and Visualize SRT "/11("r_CPratt ")
  Capture Point Computer/8(r_icp) -> "Dump and Visualize SRT "/12(r_icp)
  Capture Point Computer/9(CoP_ref) -> "Dump and Visualize SRT "/13(COPref), "CoP_ref "/1

== system stepRecovery/DesValues/State Machine Step Recovery/visualise inertial/Visualize hom transf1 ==
  H : Inport
  "CoM6D ->  CoMXYZ1" : Selector  NumberOfDimensions=2  InputPortWidth=7  IndexOptions=Index vector (dialog),Index vector (dialog)  Indices=[1 2 3],[1 2 3]  OutputSizes=1,1
  "CoM6D ->  CoMXYZ2" : Selector  NumberOfDimensions=2  InputPortWidth=7  IndexOptions=Index vector (dialog),Index vector (dialog)  Indices=[1 2 3],[4]  OutputSizes=1,1
  Hom : Scope
  MATLAB Function : MATLAB Function  TreatAsAtomicUnit=on
  p : Scope
  rollPitchYaw : Scope
  wires:
  MATLAB Function/1(rollPitchYaw) -> rollPitchYaw/1
  "CoM6D ->  CoMXYZ1"/1 -> MATLAB Function/1(R)
  H/1 -> "CoM6D ->  CoMXYZ1"/1, Hom/1, "CoM6D ->  CoMXYZ2"/1
  "CoM6D ->  CoMXYZ2"/1 -> p/1

== system stepRecovery/DesValues/State Machine Step Recovery/visualise inertial/Visualize hom transf2 ==
  H : Inport
  "CoM6D ->  CoMXYZ1" : Selector  NumberOfDimensions=2  InputPortWidth=7  IndexOptions=Index vector (dialog),Index vector (dialog)  Indices=[1 2 3],[1 2 3]  OutputSizes=1,1
  "CoM6D ->  CoMXYZ2" : Selector  NumberOfDimensions=2  InputPortWidth=7  IndexOptions=Index vector (dialog),Index vector (dialog)  Indices=[1 2 3],[4]  OutputSizes=1,1
  Hom : Scope
  MATLAB Function : MATLAB Function  TreatAsAtomicUnit=on
  p : Scope
  rollPitchYaw : Scope
  wires:
  MATLAB Function/1(rollPitchYaw) -> rollPitchYaw/1
  "CoM6D ->  CoMXYZ1"/1 -> MATLAB Function/1(R)
  H/1 -> "CoM6D ->  CoMXYZ1"/1, Hom/1, "CoM6D ->  CoMXYZ2"/1
  "CoM6D ->  CoMXYZ2"/1 -> p/1

== system stepRecovery/DesValues/State Machine Step Recovery/visualise inertial/Visualize hom transf3 ==
  H : Inport
  "CoM6D ->  CoMXYZ1" : Selector  NumberOfDimensions=2  InputPortWidth=7  IndexOptions=Index vector (dialog),Index vector (dialog)  Indices=[1 2 3],[1 2 3]  OutputSizes=1,1
  "CoM6D ->  CoMXYZ2" : Selector  NumberOfDimensions=2  InputPortWidth=7  IndexOptions=Index vector (dialog),Index vector (dialog)  Indices=[1 2 3],[4]  OutputSizes=1,1
  Hom : Scope
  MATLAB Function : MATLAB Function  TreatAsAtomicUnit=on
  p : Scope
  rollPitchYaw : Scope
  wires:
  MATLAB Function/1(rollPitchYaw) -> rollPitchYaw/1
  "CoM6D ->  CoMXYZ1"/1 -> MATLAB Function/1(R)
  H/1 -> "CoM6D ->  CoMXYZ1"/1, Hom/1, "CoM6D ->  CoMXYZ2"/1
  "CoM6D ->  CoMXYZ2"/1 -> p/1

== system stepRecovery/DesValues/State Machine Step Recovery/visualise inertial/Visualize hom transf4 ==
  H : Inport
  "CoM6D ->  CoMXYZ1" : Selector  NumberOfDimensions=2  InputPortWidth=7  IndexOptions=Index vector (dialog),Index vector (dialog)  Indices=[1 2 3],[1 2 3]  OutputSizes=1,1
  "CoM6D ->  CoMXYZ2" : Selector  NumberOfDimensions=2  InputPortWidth=7  IndexOptions=Index vector (dialog),Index vector (dialog)  Indices=[1 2 3],[4]  OutputSizes=1,1
  Hom : Scope
  MATLAB Function : MATLAB Function  TreatAsAtomicUnit=on
  p : Scope
  rollPitchYaw : Scope
  wires:
  MATLAB Function/1(rollPitchYaw) -> rollPitchYaw/1
  "CoM6D ->  CoMXYZ1"/1 -> MATLAB Function/1(R)
  H/1 -> "CoM6D ->  CoMXYZ1"/1, Hom/1, "CoM6D ->  CoMXYZ2"/1
  "CoM6D ->  CoMXYZ2"/1 -> p/1

== system stepRecovery/DesValues/State Machine Step Recovery/visualise inertial/Visualize hom transf5 ==
  H : Inport
  "CoM6D ->  CoMXYZ1" : Selector  NumberOfDimensions=2  InputPortWidth=7  IndexOptions=Index vector (dialog),Index vector (dialog)  Indices=[1 2 3],[1 2 3]  OutputSizes=1,1
  Hom : Scope
  MATLAB Function : MATLAB Function  TreatAsAtomicUnit=on
  p : Scope
  position : Selector  NumberOfDimensions=2  InputPortWidth=7  IndexOptions=Index vector (dialog),Index vector (dialog)  Indices=[1 2 3],[4]  OutputSizes=1,1
  rollPitchYaw : Scope
  wires:
  MATLAB Function/1(rollPitchYaw) -> rollPitchYaw/1  "rollPitchYaw"
  "CoM6D ->  CoMXYZ1"/1 -> MATLAB Function/1(R)
  H/1 -> "CoM6D ->  CoMXYZ1"/1, Hom/1, position/1  "H"
  position/1 -> p/1  "position"

== system stepRecovery/DesValues/State Machine Step Recovery/visualise inertial/Visualize hom transf6 ==
  H : Inport
  "CoM6D ->  CoMXYZ1" : Selector  NumberOfDimensions=2  InputPortWidth=7  IndexOptions=Index vector (dialog),Index vector (dialog)  Indices=[1 2 3],[1 2 3]  OutputSizes=1,1
  "CoM6D ->  CoMXYZ2" : Selector  NumberOfDimensions=2  InputPortWidth=7  IndexOptions=Index vector (dialog),Index vector (dialog)  Indices=[1 2 3],[4]  OutputSizes=1,1
  Hom : Scope
  MATLAB Function : MATLAB Function  TreatAsAtomicUnit=on
  p : Scope
  rollPitchYaw : Scope
  wires:
  MATLAB Function/1(rollPitchYaw) -> rollPitchYaw/1
  "CoM6D ->  CoMXYZ1"/1 -> MATLAB Function/1(R)
  H/1 -> "CoM6D ->  CoMXYZ1"/1, Hom/1, "CoM6D ->  CoMXYZ2"/1
  "CoM6D ->  CoMXYZ2"/1 -> p/1

== system stepRecovery/DesValues/State Machine Step Recovery/visualise inertial/l_sole_H_root_link2 ==
  qj : Inport
  Constant5 : Constant  Value=eye(4)
  Constant6 : Constant  Value=eye(4)
  Inv\* : Product  Inputs=/*  Multiplication=Matrix(*)
  Visualize hom transf4 : Subsystem
  link_name : WBToolboxLibrary/wholeBodyModel/Kinematics/Forward Kinematics  frameName=link_name  robotName=WBT_robotName  localName=WBT_modelName  wbiFile=WBT_wbiFilename  wbiList=WBT_wbiList
  root_link : WBToolboxLibrary/wholeBodyModel/Kinematics/Forward Kinematics  frameName='root_link'  robotName=WBT_robotName  localName=WBT_modelName  wbiFile=WBT_wbiFilename  wbiList=WBT_wbiList
  link_name_H_root_link : Outport
  wires:
  root_link/1 -> Inv\*/2, Visualize hom transf4/1(H)
  qj/1 -> root_link/2, link_name/2
  Constant6/1 -> root_link/1
  link_name/1 -> Inv\*/1
  Inv\*/1 -> link_name_H_root_link/1  "link_name_H_root_link"
  Constant5/1 -> link_name/1

== system stepRecovery/DesValues/State Machine Step Recovery/visualise inertial/l_sole_H_root_link3 ==
  qj : Inport
  Constant5 : Constant  Value=eye(4)
  Constant6 : Constant  Value=eye(4)
  Inv\* : Product  Inputs=/*  Multiplication=Matrix(*)
  Visualize hom transf4 : Subsystem
  link_name : WBToolboxLibrary/wholeBodyModel/Kinematics/Forward Kinematics  frameName=link_name  robotName=WBT_robotName  localName=WBT_modelName  wbiFile=WBT_wbiFilename  wbiList=WBT_wbiList
  root_link : WBToolboxLibrary/wholeBodyModel/Kinematics/Forward Kinematics  frameName='root_link'  robotName=WBT_robotName  localName=WBT_modelName  wbiFile=WBT_wbiFilename  wbiList=WBT_wbiList
  link_name_H_root_link : Outport
  wires:
  root_link/1 -> Inv\*/2, Visualize hom transf4/1(H)
  qj/1 -> root_link/2, link_name/2
  Constant6/1 -> root_link/1
  link_name/1 -> Inv\*/1
  Inv\*/1 -> link_name_H_root_link/1  "link_name_H_root_link"
  Constant5/1 -> link_name/1

== system stepRecovery/DesValues/State Machine Step Recovery/visualise inertial/w_H_root_link1 ==
  qj : Inport
  inertial : Inport  Port=2
  "CoM6D ->  CoMXYZ1" : Selector  NumberOfDimensions=2  InputPortWidth=7  IndexOptions=Index vector (dialog),Index vector (dialog)  Indices=[1 2 3],[1 2 3]  OutputSizes=1,1
  Constant : Constant  Value=zeros(3,1)
  Constant2 : Constant  Value=eye(4)
  Constant5 : Constant  Value=eye(4)
  Constant6 : Constant  Value=eye(4)
  Gain : Gain  Gain=pi/180
  Head state : WBToolboxLibrary/Utilities/Yarp Read  portName=[WBT_robotName, '/head/state:o']  signalSize=6  blocking=off  timestamp=off  autoconnect=on  errorOnConnection=off
  Inv\* : Product  Inputs=/*  Multiplication=Matrix(*)
  Inv\*1 : Product  Inputs=/*  Multiplication=Matrix(*)
  Inv\*2 : Product  Inputs=/  Multiplication=Matrix(*)
  Product : Product  Multiplication=Matrix(*)
  Selector : Selector  InputPortWidth=12  IndexOptions=Index vector (dialog)  Indices=[4 5 6 ]  OutputSizes=1
  Selector1 : Selector  InputPortWidth=6  IndexOptions=Index vector (dialog)  Indices=[1:3]  OutputSizes=1
  Switch : Switch  Criteria=u2 > Threshold
  Switch6 : Switch  Criteria=u2 > Threshold
  USE_IMU4EST_BASE : Constant  Value=CONFIG.USE_IMU4EST_BASE
  USE_IMU4EST_BASE1 : Constant  Value=CONFIG.CORRECT_NECK_IMU
  fromImuToHomogeousTransformFCN : MATLAB Function  TreatAsAtomicUnit=on
  holder 1 : WBToolboxLibrary/Utilities/holder 
  holder 2 : WBToolboxLibrary/Utilities/holder 
  imu : WBToolboxLibrary/wholeBodyModel/Kinematics/Forward Kinematics  frameName='imu_frame'  robotName=WBT_robotName  localName=WBT_modelName  wbiFile=WBT_wbiFilename  wbiList=WBT_wbiList
  l_sole_acc : Scope
  link : WBToolboxLibrary/wholeBodyModel/Kinematics/Forward Kinematics  frameName=link_name  robotName=WBT_robotName  localName=WBT_modelName  wbiFile=WBT_wbiFilename  wbiList=WBT_wbiList
  root_link : WBToolboxLibrary/wholeBodyModel/Kinematics/Forward Kinematics  frameName='root_link'  robotName=WBT_robotName  localName=WBT_modelName  wbiFile=WBT_wbiFilename  wbiList=WBT_wbiList
  w_H_root : Outport
  wires:
  Constant/1 -> Switch/3
  Gain/1 -> Selector1/1
  Switch/1 -> fromImuToHomogeousTransformFCN/6(neck)
  USE_IMU4EST_BASE1/1 -> Switch/2
  Selector1/1 -> Switch/1  "neck"
  Head state/1 -> Gain/1
  Product/1 -> l_sole_acc/1
  Selector/1 -> Product/2  "imu_acce"
  "CoM6D ->  CoMXYZ1"/1 -> Product/1  "l_sole_R_imu"
  Inv\*2/1 -> "CoM6D ->  CoMXYZ1"/1
  holder 2/1 -> fromImuToHomogeousTransformFCN/4(inertial_0)
  holder 1/1 -> fromImuToHomogeousTransformFCN/2(imu_H_link_0)
  root_link/1 -> Inv\*1/2
  qj/1 -> imu/2, link/2, root_link/2
  Constant2/1 -> root_link/1
  fromImuToHomogeousTransformFCN/1(w_H_root) -> Switch6/1
  USE_IMU4EST_BASE/1 -> Switch6/2
  Switch6/1 -> w_H_root/1
  inertial/1 -> fromImuToHomogeousTransformFCN/5(inertial), holder 2/1, Selector/1
  link/1 -> Inv\*1/1, Inv\*/2
  Inv\*1/1 -> fromImuToHomogeousTransformFCN/3(link_H_root), Switch6/3  "link_H_root"
  Constant6/1 -> link/1
  imu/1 -> Inv\*/1
  Inv\*/1 -> fromImuToHomogeousTransformFCN/1(imu_H_link), holder 1/1, Inv\*2/1  "imu_H_link"
  Constant5/1 -> imu/1

== system stepRecovery/DesValues/State Machine Step Recovery/visualise inertial/w_H_root_link4 ==
  qj : Inport
  inertial : Inport  Port=2
  "CoM6D ->  CoMXYZ1" : Selector  NumberOfDimensions=2  InputPortWidth=7  IndexOptions=Index vector (dialog),Index vector (dialog)  Indices=[1 2 3],[1 2 3]  OutputSizes=1,1
  Constant : Constant  Value=zeros(3,1)
  Constant2 : Constant  Value=eye(4)
  Constant5 : Constant  Value=eye(4)
  Constant6 : Constant  Value=eye(4)
  Gain : Gain  Gain=pi/180
  Head state : WBToolboxLibrary/Utilities/Yarp Read  portName=[WBT_robotName, '/head/state:o']  signalSize=6  blocking=off  timestamp=off  autoconnect=on  errorOnConnection=off
  Inv\* : Product  Inputs=/*  Multiplication=Matrix(*)
  Inv\*1 : Product  Inputs=/*  Multiplication=Matrix(*)
  Inv\*2 : Product  Inputs=/  Multiplication=Matrix(*)
  Product : Product  Multiplication=Matrix(*)
  Selector : Selector  InputPortWidth=12  IndexOptions=Index vector (dialog)  Indices=[4 5 6 ]  OutputSizes=1
  Selector1 : Selector  InputPortWidth=6  IndexOptions=Index vector (dialog)  Indices=[1:3]  OutputSizes=1
  Switch : Switch  Criteria=u2 > Threshold
  Switch6 : Switch  Criteria=u2 > Threshold
  USE_IMU4EST_BASE : Constant  Value=CONFIG.USE_IMU4EST_BASE
  USE_IMU4EST_BASE1 : Constant  Value=CONFIG.CORRECT_NECK_IMU
  fromImuToHomogeousTransformFCN : MATLAB Function  TreatAsAtomicUnit=on
  holder 1 : WBToolboxLibrary/Utilities/holder 
  holder 2 : WBToolboxLibrary/Utilities/holder 
  imu : WBToolboxLibrary/wholeBodyModel/Kinematics/Forward Kinematics  frameName='imu_frame'  robotName=WBT_robotName  localName=WBT_modelName  wbiFile=WBT_wbiFilename  wbiList=WBT_wbiList
  l_sole_acc : Scope
  link : WBToolboxLibrary/wholeBodyModel/Kinematics/Forward Kinematics  frameName=link_name  robotName=WBT_robotName  localName=WBT_modelName  wbiFile=WBT_wbiFilename  wbiList=WBT_wbiList
  root_link : WBToolboxLibrary/wholeBodyModel/Kinematics/Forward Kinematics  frameName='root_link'  robotName=WBT_robotName  localName=WBT_modelName  wbiFile=WBT_wbiFilename  wbiList=WBT_wbiList
  w_H_root : Outport
  wires:
  Constant/1 -> Switch/3
  Gain/1 -> Selector1/1
  Switch/1 -> fromImuToHomogeousTransformFCN/6(neck)
  USE_IMU4EST_BASE1/1 -> Switch/2
  Selector1/1 -> Switch/1  "neck"
  Head state/1 -> Gain/1
  Product/1 -> l_sole_acc/1
  Selector/1 -> Product/2  "imu_acce"
  "CoM6D ->  CoMXYZ1"/1 -> Product/1  "l_sole_R_imu"
  Inv\*2/1 -> "CoM6D ->  CoMXYZ1"/1
  holder 2/1 -> fromImuToHomogeousTransformFCN/4(inertial_0)
  holder 1/1 -> fromImuToHomogeousTransformFCN/2(imu_H_link_0)
  root_link/1 -> Inv\*1/2
  qj/1 -> imu/2, link/2, root_link/2
  Constant2/1 -> root_link/1
  fromImuToHomogeousTransformFCN/1(w_H_root) -> Switch6/1
  USE_IMU4EST_BASE/1 -> Switch6/2
  Switch6/1 -> w_H_root/1
  inertial/1 -> fromImuToHomogeousTransformFCN/5(inertial), holder 2/1, Selector/1
  link/1 -> Inv\*1/1, Inv\*/2
  Inv\*1/1 -> fromImuToHomogeousTransformFCN/3(link_H_root), Switch6/3  "link_H_root"
  Constant6/1 -> link/1
  imu/1 -> Inv\*/1
  Inv\*/1 -> fromImuToHomogeousTransformFCN/1(imu_H_link), holder 1/1, Inv\*2/1  "imu_H_link"
  Constant5/1 -> imu/1

== system stepRecovery/DesValues/State Machine Step Recovery/Step Recovery reference generator/Inverse Kinematics/NL_IK ==
  qj(0) : Inport
  w_H_b : Inport  Port=2
  Desired Transformation : Inport  Port=3
  Enable : EnablePort  StatesWhenEnabling=reset
  Constant : Constant  Value=CONFIG.useLocalIK
  Constant1 : Constant  Value=CONFIG.useLocalIK
  Data Type Conversion : DataTypeConversion  OutDataTypeStr=boolean
  Demux : Demux  Outputs=[12,1,ROBOT_DOF]
  Local Inverse Kinematics : Subsystem
  Logical Operator : Logic  Operator=NOT  AllPortsSameDT=off  OutDataTypeStr=boolean
  Mux : Mux  Inputs=3
  Mux1 : Mux  Inputs=3
  Remote Inverse Kinematics : Subsystem
  Switch : Switch  Criteria=u2 > Threshold
  OUT : Outport
  q_legs : Outport  Port=2
  q_total : Outport  Port=3
  wires:
  qj(0)/1 -> Remote Inverse Kinematics/1(q(0)), Local Inverse Kinematics/3(qj(0))
  Desired Transformation/1 -> Remote Inverse Kinematics/2("Desired Transformation "), Local Inverse Kinematics/1(Desired Transformation)
  w_H_b/1 -> Local Inverse Kinematics/2(w_H_b)
  Constant/1 -> Logical Operator/1, Local Inverse Kinematics/Enable
  Logical Operator/1 -> Remote Inverse Kinematics/Enable
  Local Inverse Kinematics/2(OUT) -> Mux/2
  Local Inverse Kinematics/1(q_legs) -> Mux/1
  Local Inverse Kinematics/3(q_total) -> Mux/3
  Remote Inverse Kinematics/1(q_legs) -> Mux1/1
  Remote Inverse Kinematics/2(OUT) -> Mux1/2
  Remote Inverse Kinematics/3(q_total) -> Mux1/3
  Mux/1 -> Switch/1
  Mux1/1 -> Switch/3
  Constant1/1 -> Switch/2
  Switch/1 -> Demux/1
  Demux/1 -> q_legs/1
  Demux/2 -> Data Type Conversion/1
  Demux/3 -> q_total/1
  Data Type Conversion/1 -> OUT/1
